simulink model "YoulaSwitch"  (R2019b)
settings: Solver=ode4  StartTime=0.0  StopTime=10  FixedStep=1e-3  MaxStep=0.01  RelTol=1e-4  EnableMultiTasking=on
values from neighbouring files (symbols this model uses):
  K1 = ss(zeros(ncont,nmeas,3))    [Demo_007.m]    (also in Demo_012.m = ss(tf([Kp1,Ki1],[1 0])))
  K2 = ss(zeros(ncont,nmeas,3))    [Demo_007.m]    (also in Demo_012.m = ss(tf([Kp2,Ki2],[1 0])))
  mode = nu    [Demo_012.m]
  olic = sysic    [Demo_003.m]    (also in Demo_009.m; Demo_012.m = Usamp(:,:,i,1); Demo_014.m; Demo_015.m)
  Q1 = Q{1}    [Demo_012.m]
  Q2 = Q{2}    [Demo_012.m]
undefined symbols (not defined in the file or in its folder): L, nKi, nKo, nQi, nQo
libraries: simulink x1
settings Model: Creator=Joost Veenman  LastModifiedBy=joost.veenman
settings DataIOCC: LimitDataPoints=on  SaveFormat=Array  SignalLoggingSaveFormat=ModelDataLogs  ReturnWorkspaceOutputs=off
settings OptimizationCC: ExpressionDepthLimit=2147483647  InitFltsAndDblsToZero=on  LifeSpan=inf
settings DebuggingCC: AlgebraicLoopMsg=none  UnderspecifiedInitializationDetection=Classic  MergeDetectMultiDrivingBlocksExec=none  SolverPrmCheckMsg=warning  FcnCallInpInsideContextMsg=warning  StateNameClashWarn=warning  SFUnexpectedBacktrackingDiag=warning  SFNoUnconditionalDefaultTransitionDiag=warning  SFExecutionAtInitializationDiag=none  ArithmeticOperatorsInVariantConditions=warning
settings HardwareCC: ProdBitPerPointer=32  ProdBitPerSizeT=32  ProdBitPerPtrDiffT=32  ProdLargestAtomicFloat=None  ProdIntDivRoundTo=Undefined  ProdEndianess=Unspecified  ProdWordSize=32  ProdHWDeviceType=32-bit Generic
settings ModelReferenceCC: PropagateSignalLabelsOutOfModel=off
settings SFSimCC: SimUseLocalCustomCode=off  SimParseCustomCode=off  CustomCodeUndefinedFunction=UseInterfaceOnly
settings RTWCC: RTWUseLocalCustomCode=off
settings CodeAppCC: StateflowObjectComments=on
settings GRTTargetCC: TargetLangStandard=C89/C90 (ANSI)  GeneratePreprocessorConditionals=Disable all  CombineOutputUpdateFcns=off  GRTInterface=on
settings ConfigComp: CovMetricSettings=dw  CovHtmlReporting=on  CovSaveCumulativeToWorkspaceVar=on  CovSaveSingleToWorkspaceVar=on  CovExternalEMLEnable=off

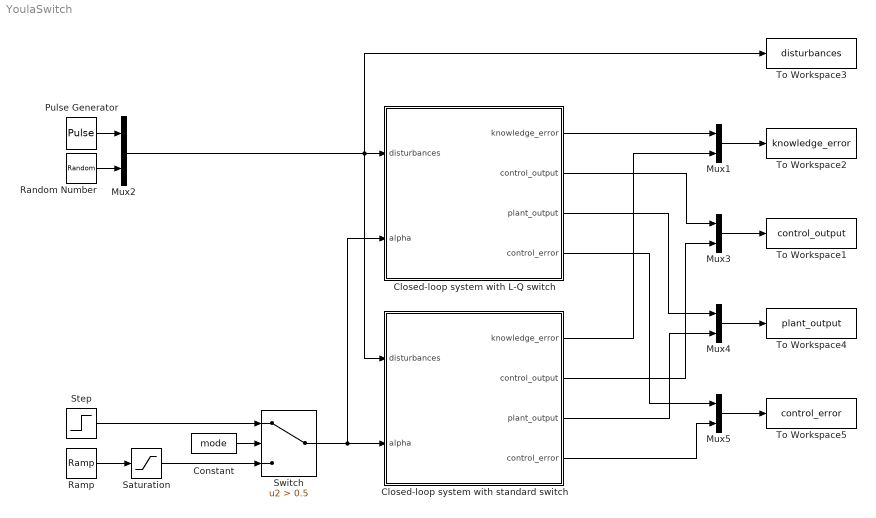
== system YoulaSwitch ==
  Closed-loop system with L-Q switch : Subsystem
  Closed-loop system with standard switch : Subsystem
  Constant : Constant  Value=mode
  Mux{1..5} (5 alike) : Mux  Inputs=2
  Pulse Generator : DiscretePulseGenerator  PulseType=Time based  Period=20  PulseWidth=30
  Ramp : simulink/Sources/Ramp  slope=0.5  start=6  InitialOutput=0
  Random Number : RandomNumber  Variance=0.01  Seed=1235  SampleTime=1e-3
  Saturation : Saturate  UpperLimit=1  LowerLimit=0
  Step : Step  Time=6  SampleTime=0
  Switch : Switch  Criteria=u2 > Threshold  Threshold=0.5
  To Workspace1 : ToWorkspace  VariableName=control_output  SaveFormat=Timeseries  SampleTime=-1
  To Workspace2 : ToWorkspace  VariableName=knowledge_error  SaveFormat=Timeseries  SampleTime=-1
  To Workspace3 : ToWorkspace  VariableName=disturbances  SaveFormat=Timeseries  SampleTime=-1
  To Workspace4 : ToWorkspace  VariableName=plant_output  SaveFormat=Timeseries  SampleTime=-1
  To Workspace5 : ToWorkspace  VariableName=control_error  SaveFormat=Timeseries  SampleTime=-1
  wires:
  Step/1 -> Switch/1
  Ramp/1 -> Saturation/1
  Saturation/1 -> Switch/3
  Switch/1 -> Closed-loop system with standard switch/2(alpha), Closed-loop system with L-Q switch/2(alpha)
  Pulse Generator/1 -> Mux2/1
  Closed-loop system with standard switch/1(knowledge_error) -> Mux1/2
  Mux2/1 -> To Workspace3/1, Closed-loop system with standard switch/1(disturbances), Closed-loop system with L-Q switch/1(disturbances)
  Random Number/1 -> Mux2/2
  Mux3/1 -> To Workspace1/1
  Closed-loop system with L-Q switch/1(knowledge_error) -> Mux1/1
  Mux1/1 -> To Workspace2/1
  Closed-loop system with L-Q switch/2(control_output) -> Mux3/1
  Closed-loop system with standard switch/2(control_output) -> Mux3/2
  Constant/1 -> Switch/2
  Mux4/1 -> To Workspace4/1
  Mux5/1 -> To Workspace5/1
  Closed-loop system with standard switch/4(control_error) -> Mux5/2
  Closed-loop system with standard switch/3(plant_output) -> Mux4/2
  Closed-loop system with L-Q switch/3(plant_output) -> Mux4/1
  Closed-loop system with L-Q switch/4(control_error) -> Mux5/1

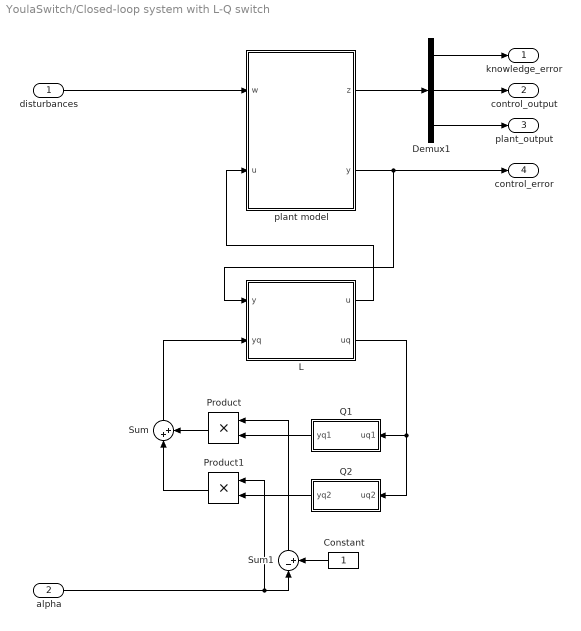
== system YoulaSwitch/Closed-loop system with L-Q switch ==
  disturbances : Inport
  alpha : Inport  Port=2
  Constant : Constant
  Demux1 : Demux  Outputs=3
  L : Subsystem
  Product : Product
  Product1 : Product
  Q1 : Subsystem
  Q2 : Subsystem
  Sum : Sum  Inputs=|++
  Sum1 : Sum  Inputs=|-+
  plant model : Subsystem
  knowledge_error : Outport
  control_output : Outport  Port=2
  plant_output : Outport  Port=3
  control_error : Outport  Port=4
  wires:
  Constant/1 -> Sum1/2
  alpha/1 -> Sum1/1, Product1/1
  L/2(uq) -> Q2/1(uq2), Q1/1(uq1)
  plant model/2(y) -> L/1(y), control_error/1
  Q2/1(yq2) -> Product1/2
  L/1(u) -> plant model/2(u)
  Product1/1 -> Sum/1
  Q1/1(yq1) -> Product/2
  Sum1/1 -> Product/1
  Product/1 -> Sum/2
  Sum/1 -> L/2(yq)
  disturbances/1 -> plant model/1(w)
  plant model/1(z) -> Demux1/1
  Demux1/1 -> knowledge_error/1
  Demux1/2 -> control_output/1
  Demux1/3 -> plant_output/1

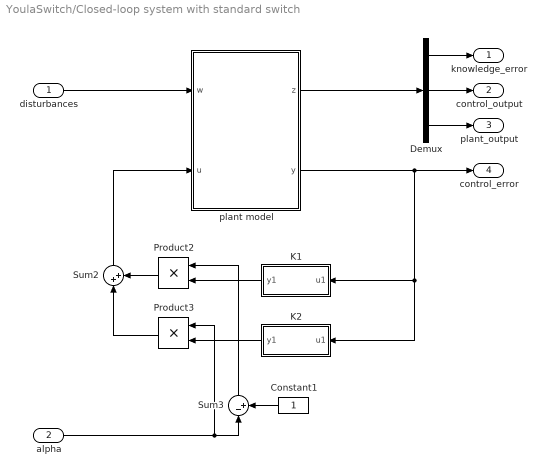
== system YoulaSwitch/Closed-loop system with standard switch ==
  disturbances : Inport
  alpha : Inport  Port=2
  Constant1 : Constant
  Demux : Demux  Outputs=3
  K1 : Subsystem
  K2 : Subsystem
  Product2 : Product
  Product3 : Product
  Sum2 : Sum  Inputs=|++
  Sum3 : Sum  Inputs=|-+
  plant model : Subsystem
  knowledge_error : Outport
  control_output : Outport  Port=2
  plant_output : Outport  Port=3
  control_error : Outport  Port=4
  wires:
  disturbances/1 -> plant model/1(w)
  Demux/2 -> control_output/1
  plant model/1(z) -> Demux/1
  Demux/1 -> knowledge_error/1
  Sum3/1 -> Product2/1
  K1/1(y1) -> Product2/2
  Product3/1 -> Sum2/1
  plant model/2(y) -> K2/1(u1), K1/1(u1), control_error/1
  Constant1/1 -> Sum3/2
  Product2/1 -> Sum2/2
  Sum2/1 -> plant model/2(u)
  K2/1(y1) -> Product3/2
  alpha/1 -> Sum3/1, Product3/1
  Demux/3 -> plant_output/1

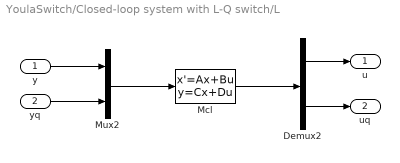
== system YoulaSwitch/Closed-loop system with L-Q switch/L ==
  y : Inport
  yq : Inport  Port=2
  Demux2 : Demux  Outputs=[nKo,nQi]
  Mcl : StateSpace  A=L.a  B=L.b  C=L.c  D=L.d  InitialCondition=0
  Mux2 : Mux  Inputs=[nKi,nQo]
  u : Outport
  uq : Outport  Port=2
  wires:
  Demux2/1 -> u/1
  Demux2/2 -> uq/1
  y/1 -> Mux2/1
  yq/1 -> Mux2/2
  Mux2/1 -> Mcl/1
  Mcl/1 -> Demux2/1

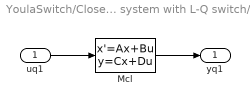
== system YoulaSwitch/Closed-loop system with L-Q switch/Q1 ==
  uq1 : Inport
  Mcl : StateSpace  A=Q1.a  B=Q1.b  C=Q1.c  D=Q1.d  InitialCondition=0
  yq1 : Outport
  wires:
  Mcl/1 -> yq1/1
  uq1/1 -> Mcl/1

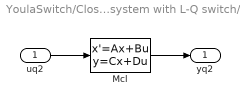
== system YoulaSwitch/Closed-loop system with L-Q switch/Q2 ==
  uq2 : Inport
  Mcl : StateSpace  A=Q2.a  B=Q2.b  C=Q2.c  D=Q2.d  InitialCondition=0
  yq2 : Outport
  wires:
  uq2/1 -> Mcl/1
  Mcl/1 -> yq2/1

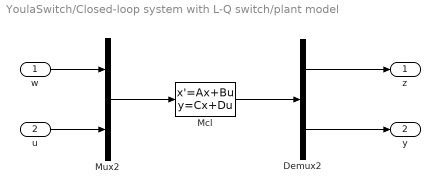
== system YoulaSwitch/Closed-loop system with L-Q switch/plant model ==
  w : Inport
  u : Inport  Port=2
  Demux2 : Demux  Outputs=[3,1]
  Mcl : StateSpace  A=olic.a  B=olic.b  C=olic.c  D=olic.d  InitialCondition=0
  Mux2 : Mux  Inputs=[2,1]
  z : Outport
  y : Outport  Port=2
  wires:
  Demux2/1 -> z/1
  u/1 -> Mux2/2
  Mux2/1 -> Mcl/1
  Mcl/1 -> Demux2/1
  Demux2/2 -> y/1
  w/1 -> Mux2/1

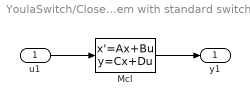
== system YoulaSwitch/Closed-loop system with standard switch/K1 ==
  u1 : Inport
  Mcl : StateSpace  A=K1.a  B=K1.b  C=K1.c  D=K1.d  InitialCondition=0
  y1 : Outport
  wires:
  Mcl/1 -> y1/1
  u1/1 -> Mcl/1

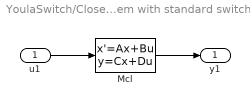
== system YoulaSwitch/Closed-loop system with standard switch/K2 ==
  u1 : Inport
  Mcl : StateSpace  A=K2.a  B=K2.b  C=K2.c  D=K2.d  InitialCondition=0
  y1 : Outport
  wires:
  Mcl/1 -> y1/1
  u1/1 -> Mcl/1

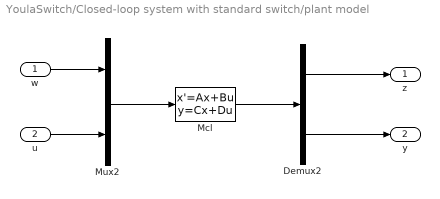
== system YoulaSwitch/Closed-loop system with standard switch/plant model ==
  w : Inport
  u : Inport  Port=2
  Demux2 : Demux  Outputs=[3,1]
  Mcl : StateSpace  A=olic.a  B=olic.b  C=olic.c  D=olic.d  InitialCondition=0
  Mux2 : Mux  Inputs=[2,1]
  z : Outport
  y : Outport  Port=2
  wires:
  Mcl/1 -> Demux2/1
  Demux2/1 -> z/1
  u/1 -> Mux2/2
  Mux2/1 -> Mcl/1
  Demux2/2 -> y/1
  w/1 -> Mux2/1
